simulink model "SeriesPHEV_New_Test2"  (R2018a)
settings: Solver=ode4  StartTime=0.0  StopTime=1367  FixedStep=0.01  RelTol=1e-3  EnableMultiTasking=on
undefined symbols (not defined in the file): cells, Eff, engine_rad, ES_dem, FDR, ftp, GT, InitialSOC, mdot, MG_dem, MGS, MT, P_ice, P_ice_dem, Regen, SOC_ICE, T_dem, tau_engine, throttle, time, Torq
settings Model: Creator=Administrator  LastModifiedBy=user2
settings DataIOCC: LimitDataPoints=on  SaveFormat=Array  SignalLoggingSaveFormat=ModelDataLogs
settings OptimizationCC: ExpressionDepthLimit=2147483647  LifeSpan=inf
settings DebuggingCC: UnderspecifiedInitializationDetection=Classic  MergeDetectMultiDrivingBlocksExec=none  SolverPrmCheckMsg=warning  FcnCallInpInsideContextMsg=warning  StateNameClashWarn=warning  SFUnexpectedBacktrackingDiag=warning  SFNoUnconditionalDefaultTransitionDiag=warning  SFExecutionAtInitializationDiag=none
settings HardwareCC: ProdBitPerPointer=32  ProdBitPerSizeT=32  ProdBitPerPtrDiffT=32  ProdLargestAtomicFloat=None  ProdIntDivRoundTo=Undefined  ProdEndianess=Unspecified  ProdWordSize=32  ProdHWDeviceType=32-bit Generic
settings ModelReferenceCC: PropagateSignalLabelsOutOfModel=off
settings CodeAppCC: StateflowObjectComments=on
settings GRTTargetCC: TargetLangStandard=C89/C90 (ANSI)  GeneratePreprocessorConditionals=Disable all  CombineOutputUpdateFcns=off  GRTInterface=on
settings ConfigComp: CovMetricSettings=dw  CovHtmlReporting=on  CovSaveCumulativeToWorkspaceVar=on  CovSaveSingleToWorkspaceVar=on  CovExternalEMLEnable=off

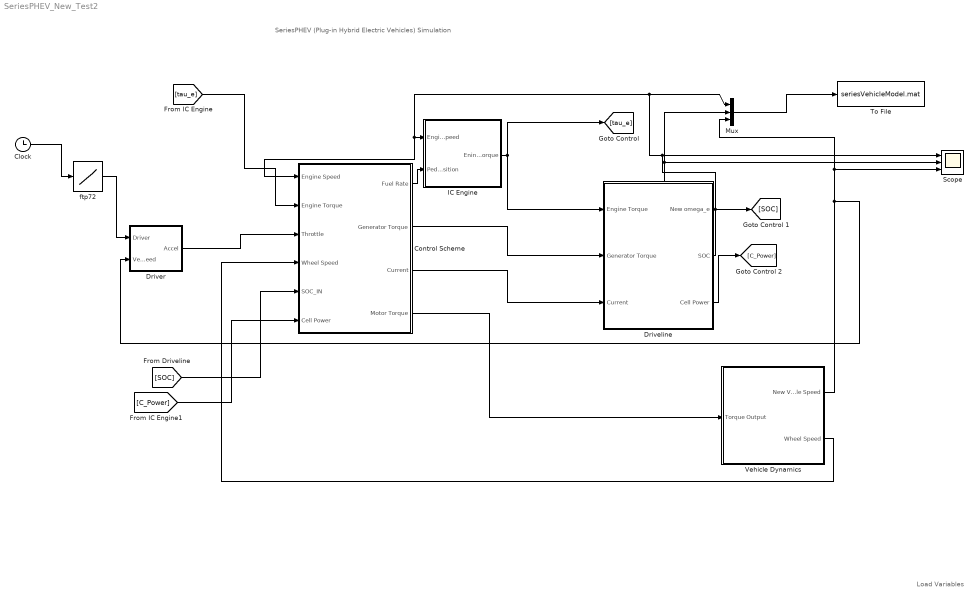
== system SeriesPHEV_New_Test2 ==
  note: SeriesPHEV (Plug-in Hybrid Electric Vehicles) Simulation
  note: Load Variables
  Clock : Clock
      settings: Decimation=100
  Control Scheme : Subsystem
  Driveline : Subsystem
  Driver : Subsystem
  IC Engine : Subsystem
  Mux : Mux  Inputs=3
  Scope : Scope  NumInputPorts=3
  To File : ToFile  Filename=seriesVehicleModel.mat  MatrixName=dynamics
  Vehicle Dynamics : Subsystem
  ftp72 : Lookup_n-D  NumberOfTableDimensions=1  BreakpointsForDimension1=time  Table=ftp  RndMeth=Simplest  InputSameDT=on
  wires:
  Mux/1 -> To File/1
  Driver/1(Accel) -> Control Scheme/3(Throttle)
  [SOC] -> Control Scheme/5(SOC_IN)
  Control Scheme/1(Fuel Rate) -> IC Engine/2(Pedal Position)
  IC Engine/1(Eninge Torque) -> [tau_e], Driveline/1(Engine Torque)
  Control Scheme/2(Generator Torque) -> Driveline/2(Generator Torque)
  Driveline/1(New omega_e) -> Mux/1, Control Scheme/1(Engine Speed), IC Engine/1(Engine Speed), Scope/1
  [tau_e] -> Control Scheme/2(Engine Torque)
  Vehicle Dynamics/1(New Vehicle Speed) -> Mux/3, Scope/3, Driver/2(Vehicle Speed)
  Vehicle Dynamics/2(Wheel Speed) -> Control Scheme/4(Wheel Speed)
  ftp72/1 -> Driver/1(Driver)
  Clock/1 -> ftp72/1
  Control Scheme/4(Motor Torque) -> Vehicle Dynamics/1(Torque Output)
  Driveline/2(SOC) -> Mux/2, Scope/2, [SOC]
  Control Scheme/3(Current) -> Driveline/3(Current)
  [C_Power] -> Control Scheme/6(Cell Power)
  Driveline/3(Cell Power) -> [C_Power]

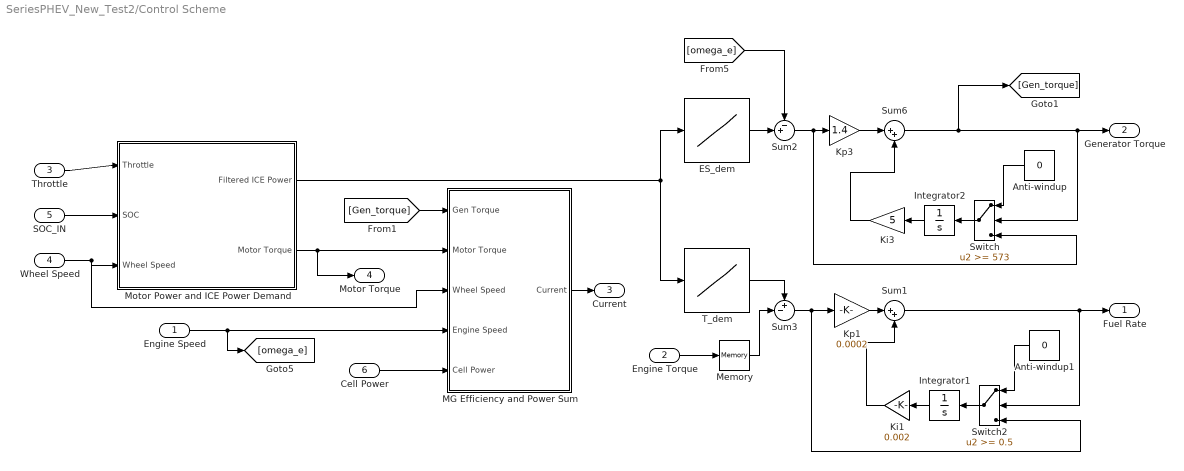
== system SeriesPHEV_New_Test2/Control Scheme ==
  Engine Speed : Inport
  Engine Torque : Inport  Port=2
  Throttle : Inport  Port=3
  Wheel Speed : Inport  Port=4
  SOC_IN : Inport  Port=5
  Cell Power : Inport  Port=6
  Anti-windup : Constant  Value=0
  Anti-windup1 : Constant  Value=0
  ES_dem : Lookup_n-D  NumberOfTableDimensions=1  BreakpointsForDimension1=P_ice  Table=ES_dem  RndMeth=Simplest  InputSameDT=on
  Integrator1 : Integrator
  Integrator2 : Integrator
  Ki1 : Gain  Gain=0.002
  Ki3 : Gain  Gain=5
  Kp1 : Gain  Gain=0.0002
  Kp3 : Gain  Gain=1.4
  MG Efficiency and Power Sum : Subsystem
  Memory : Memory  InheritSampleTime=on
  "Motor Power and ICE Power Demand " : Subsystem
  Sum1 : Sum  Inputs=|++
  Sum2 : Sum  Inputs=-+|
  Sum3 : Sum  Inputs=+-|
  Sum6 : Sum  Inputs=|++
  Switch : Switch  Threshold=573
  Switch2 : Switch  Threshold=0.5
  T_dem : Lookup_n-D  NumberOfTableDimensions=1  BreakpointsForDimension1=P_ice  Table=T_dem  RndMeth=Simplest  InputSameDT=on
  Fuel Rate : Outport
  Generator Torque : Outport  Port=2
  Current : Outport  Port=3
  Motor Torque : Outport  Port=4
  wires:
  ES_dem/1 -> Sum2/2
  T_dem/1 -> Sum3/1
  Engine Torque/1 -> Memory/1
  Kp3/1 -> Sum6/1
  Sum6/1 -> Generator Torque/1, Switch/2, [Gen_torque]
  Sum1/1 -> Fuel Rate/1, Switch2/2
  Memory/1 -> Sum3/2
  Switch/1 -> Integrator2/1
  Integrator2/1 -> Ki3/1
  Ki3/1 -> Sum6/2
  Sum2/1 -> Switch/3, Kp3/1
  Anti-windup/1 -> Switch/1
  Sum3/1 -> Kp1/1, Switch2/3
  Kp1/1 -> Sum1/1
  Switch2/1 -> Integrator1/1
  Integrator1/1 -> Ki1/1
  Ki1/1 -> Sum1/2
  Anti-windup1/1 -> Switch2/1
  MG Efficiency and Power Sum/1(Current) -> Current/1
  Cell Power/1 -> MG Efficiency and Power Sum/5(Cell Power)
  Throttle/1 -> "Motor Power and ICE Power Demand "/1(Throttle)
  SOC_IN/1 -> "Motor Power and ICE Power Demand "/2(SOC)
  Wheel Speed/1 -> "Motor Power and ICE Power Demand "/3(Wheel Speed), MG Efficiency and Power Sum/3(Wheel Speed)
  "Motor Power and ICE Power Demand "/2(Motor Torque) -> Motor Torque/1, MG Efficiency and Power Sum/2(Motor Torque)
  "Motor Power and ICE Power Demand "/1(Filtered ICE Power) -> T_dem/1, ES_dem/1
  [Gen_torque] -> MG Efficiency and Power Sum/1(Gen Torque)
  [omega_e] -> Sum2/1
  Engine Speed/1 -> MG Efficiency and Power Sum/4(Engine Speed), [omega_e]

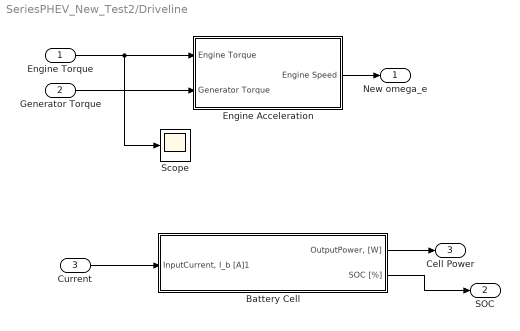
== system SeriesPHEV_New_Test2/Driveline ==
  Engine Torque : Inport
  Generator Torque : Inport  Port=2
  Current : Inport  Port=3
  Battery Cell : Subsystem
  Engine Acceleration : Subsystem
  Scope : Scope
  New omega_e : Outport
  SOC : Outport  Port=2
  Cell Power : Outport  Port=3
  wires:
  Engine Torque/1 -> Scope/1, Engine Acceleration/1(Engine Torque)
  Generator Torque/1 -> Engine Acceleration/2(Generator Torque)
  Engine Acceleration/1(Engine Speed) -> New omega_e/1
  Battery Cell/2(SOC [%]) -> SOC/1
  Current/1 -> Battery Cell/1("InputCurrent, I_b [A]1")
  Battery Cell/1("OutputPower, [W]") -> Cell Power/1

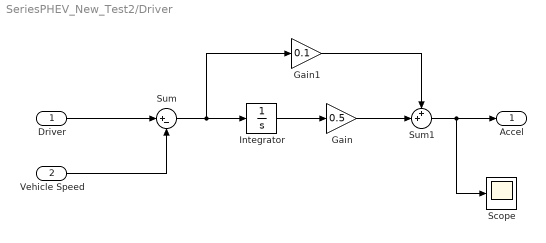
== system SeriesPHEV_New_Test2/Driver ==
  Driver : Inport
  Vehicle Speed : Inport  Port=2
  Gain : Gain  Gain=0.5
  Gain1 : Gain  Gain=0.1
  Integrator : Integrator
  Scope : Scope
  Sum : Sum  Inputs=|+-
  Sum1 : Sum  Inputs=++|
  Accel : Outport
  wires:
  Driver/1 -> Sum/1
  Vehicle Speed/1 -> Sum/2
  Sum/1 -> Integrator/1, Gain1/1
  Integrator/1 -> Gain/1
  Gain/1 -> Sum1/2
  Gain1/1 -> Sum1/1
  Sum1/1 -> Accel/1, Scope/1

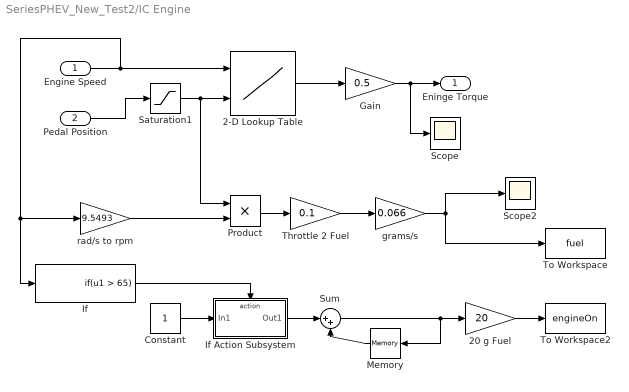
== system SeriesPHEV_New_Test2/IC Engine ==
  Engine Speed : Inport
  Pedal Position : Inport  Port=2
  2-D Lookup Table : Lookup_n-D  BreakpointsForDimension1=engine_rad  BreakpointsForDimension2=mdot  Table=tau_engine  RndMeth=Simplest  InputSameDT=on
  20 g Fuel : Gain  Gain=20
  Constant : Constant
  Gain : Gain  Gain=0.5
  If : If  IfExpression=u1 > 65  ShowElse=off
  If Action Subsystem : Subsystem  TreatAsAtomicUnit=on
  Memory : Memory
  Product : Product  RndMeth=Zero
  Saturation1 : Saturate  UpperLimit=0.4  LowerLimit=0
  Scope : Scope
  Scope2 : Scope
  Sum : Sum  Inputs=|++
  Throttle 2 Fuel : Gain  Gain=0.1
  To Workspace : ToWorkspace  VariableName=fuel  SampleTime=-1
      settings: Decimation=100
  To Workspace2 : ToWorkspace  VariableName=engineOn  SampleTime=-1
      settings: Decimation=100
  grams/s : Gain  Gain=0.066
  rad/s to rpm : Gain  Gain=9.5493
  Eninge Torque : Outport
  wires:
  Engine Speed/1 -> 2-D Lookup Table/1, rad/s to rpm/1, If/1
  Pedal Position/1 -> Saturation1/1
  Saturation1/1 -> Product/1, 2-D Lookup Table/2
  2-D Lookup Table/1 -> Gain/1
  Gain/1 -> Eninge Torque/1, Scope/1
  rad/s to rpm/1 -> Product/2
  grams/s/1 -> Scope2/1, To Workspace/1
  Memory/1 -> Sum/2
  If/1 -> If Action Subsystem/Action
  Constant/1 -> If Action Subsystem/1(In1)
  Sum/1 -> Memory/1, 20 g Fuel/1
  If Action Subsystem/1(Out1) -> Sum/1
  20 g Fuel/1 -> To Workspace2/1
  Throttle 2 Fuel/1 -> grams/s/1
  Product/1 -> Throttle 2 Fuel/1

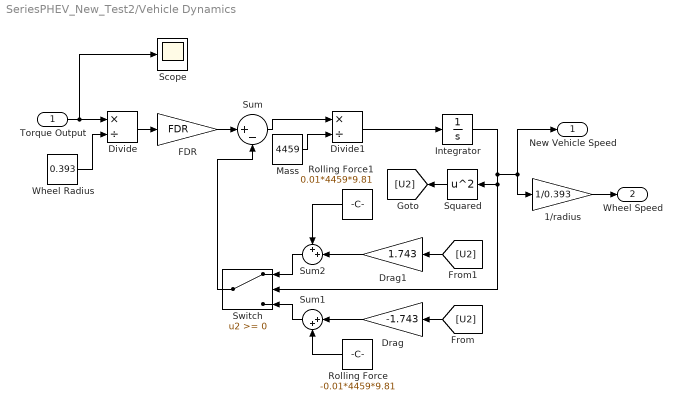
== system SeriesPHEV_New_Test2/Vehicle Dynamics ==
  Torque Output : Inport
  1/radius : Gain  Gain=1/0.393
  Divide : Product  Inputs=*/
  Divide1 : Product  Inputs=*/
  Drag : Gain  Gain=-1.743
  Drag1 : Gain  Gain=1.743
  FDR : Gain  Gain=FDR
  Integrator : Integrator
  Mass : Constant  Value=4459
  Rolling Force : Constant  Value=-0.01*4459*9.81
  Rolling Force1 : Constant  Value=0.01*4459*9.81
  Scope : Scope
  Squared : Math  Operator=square  SaturateOnIntegerOverflow=on
  Sum : Sum  Inputs=|+-
  Sum1 : Sum  Inputs=|++
  Sum2 : Sum  Inputs=++|
  Switch : Switch
  Wheel Radius : Constant  Value=0.393
  New Vehicle Speed : Outport
  Wheel Speed : Outport  Port=2
  wires:
  Torque Output/1 -> Scope/1, Divide/1
  Wheel Radius/1 -> Divide/2
  Divide/1 -> FDR/1
  1/radius/1 -> Wheel Speed/1
  Sum/1 -> Divide1/1
  Mass/1 -> Divide1/2
  Divide1/1 -> Integrator/1
  Integrator/1 -> 1/radius/1, New Vehicle Speed/1, Squared/1, Switch/2
  FDR/1 -> Sum/1
  Squared/1 -> [U2]
  Drag/1 -> Sum1/1
  Rolling Force/1 -> Sum1/2
  [U2] -> Drag/1
  Sum1/1 -> Switch/3
  [U2] -> Drag1/1
  Rolling Force1/1 -> Sum2/1
  Drag1/1 -> Sum2/2
  Sum2/1 -> Switch/1
  Switch/1 -> Sum/2

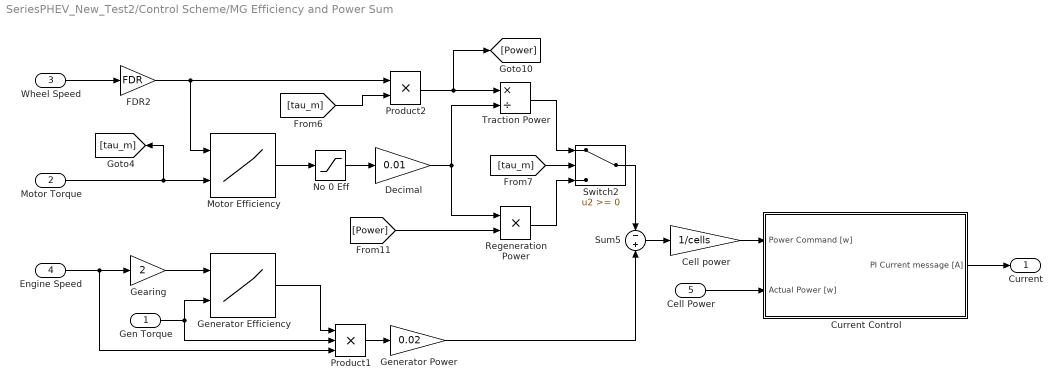
== system SeriesPHEV_New_Test2/Control Scheme/MG Efficiency and Power Sum ==
  Gen Torque : Inport
  Motor Torque : Inport  Port=2
  Wheel Speed : Inport  Port=3
  Engine Speed : Inport  Port=4
  Cell Power : Inport  Port=5
  Cell power : Gain  Gain=1/cells
  Current Control : Subsystem
  Decimal : Gain  Gain=0.01
  FDR2 : Gain  Gain=FDR
  Gearing : Gain  Gain=2
  Generator Power : Gain  Gain=0.02
  Generator Efficiency : Lookup_n-D  BreakpointsForDimension1=MGS  BreakpointsForDimension2=GT  Table=Eff  RndMeth=Simplest  InputSameDT=on
  Motor Efficiency : Lookup_n-D  BreakpointsForDimension1=MGS  BreakpointsForDimension2=MT  Table=Eff  RndMeth=Simplest  InputSameDT=on
  No 0 Eff : Saturate  UpperLimit=100  LowerLimit=0.001
  Product1 : Product  Inputs=3  RndMeth=Zero
  Product2 : Product  RndMeth=Zero
  Regeneration Power : Product  RndMeth=Zero
  Sum5 : Sum  Inputs=-+
  Switch2 : Switch
  Traction Power : Product  Inputs=*/
  Current : Outport
  wires:
  Gearing/1 -> Generator Efficiency/1
  Generator Efficiency/1 -> Product1/1
  Gen Torque/1 -> Product1/2, Generator Efficiency/2
  Product1/1 -> Generator Power/1
  Motor Efficiency/1 -> No 0 Eff/1
  [tau_m] -> Product2/2
  Product2/1 -> [Power], Traction Power/1
  Generator Power/1 -> Sum5/2
  Sum5/1 -> Cell power/1
  FDR2/1 -> Motor Efficiency/1, Product2/1
  No 0 Eff/1 -> Decimal/1
  Decimal/1 -> Regeneration Power/1, Traction Power/2
  [tau_m] -> Switch2/2
  Switch2/1 -> Sum5/1
  Regeneration Power/1 -> Switch2/3
  Traction Power/1 -> Switch2/1
  [Power] -> Regeneration Power/2
  Engine Speed/1 -> Product1/3, Gearing/1
  Motor Torque/1 -> [tau_m], Motor Efficiency/2
  Wheel Speed/1 -> FDR2/1
  Current Control/1(PI Current message [A]) -> Current/1
  Cell power/1 -> Current Control/1(Power Command [w])
  Cell Power/1 -> Current Control/2(Actual Power [w])

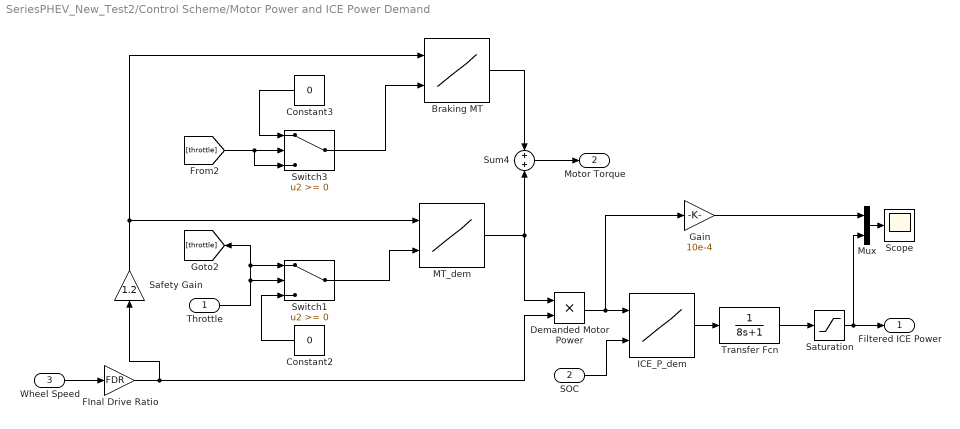
== system SeriesPHEV_New_Test2/Control Scheme/Motor Power and ICE Power Demand  ==
  Throttle : Inport
  SOC : Inport  Port=2
  Wheel Speed : Inport  Port=3
  Braking MT : Lookup_n-D  BreakpointsForDimension1=MGS  BreakpointsForDimension2=throttle  Table=Regen  RndMeth=Simplest  InputSameDT=on
  Constant2 : Constant  Value=0
  Constant3 : Constant  Value=0
  Demanded Motor Power : Product  RndMeth=Zero
  FInal Drive Ratio : Gain  Gain=FDR
  Gain : Gain  Gain=10e-4
  ICE_P_dem : Lookup_n-D  BreakpointsForDimension1=MG_dem  BreakpointsForDimension2=SOC_ICE  Table=P_ice_dem  RndMeth=Simplest  InputSameDT=on
  MT_dem : Lookup_n-D  BreakpointsForDimension1=MGS  BreakpointsForDimension2=mdot  Table=Torq  RndMeth=Simplest  InputSameDT=on
  Mux : Mux  Inputs=2
  Safety Gain : Gain  Gain=1.2
  Saturation : Saturate  UpperLimit=88.74  LowerLimit=0
  Scope : Scope
  Sum4 : Sum
  Switch1 : Switch
  Switch3 : Switch
  Transfer Fcn : TransferFcn  Denominator=[8 1]
  Filtered ICE Power : Outport
  Motor Torque : Outport  Port=2
  wires:
  FInal Drive Ratio/1 -> Demanded Motor Power/2, Safety Gain/1
  Safety Gain/1 -> MT_dem/1, Braking MT/1
  Demanded Motor Power/1 -> Gain/1, ICE_P_dem/1
  Switch1/1 -> MT_dem/2
  Constant2/1 -> Switch1/3
  Constant3/1 -> Switch3/1
  [throttle] -> Switch3/2, Switch3/3
  Switch3/1 -> Braking MT/2
  Transfer Fcn/1 -> Saturation/1
  ICE_P_dem/1 -> Transfer Fcn/1
  Braking MT/1 -> Sum4/1
  MT_dem/1 -> Sum4/2, Demanded Motor Power/1
  Wheel Speed/1 -> FInal Drive Ratio/1
  Throttle/1 -> [throttle], Switch1/1, Switch1/2
  SOC/1 -> ICE_P_dem/2
  Saturation/1 -> Mux/2, Filtered ICE Power/1
  Sum4/1 -> Motor Torque/1
  Mux/1 -> Scope/1
  Gain/1 -> Mux/1

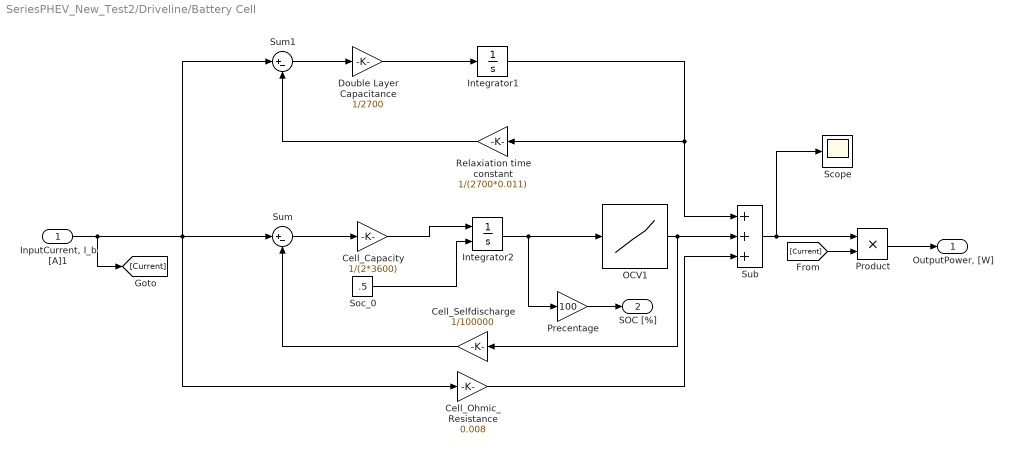
== system SeriesPHEV_New_Test2/Driveline/Battery Cell ==
  "InputCurrent, I_b [A]1" : Inport
  Cell_Capacity : Gain  Gain=1/(2*3600)
  Cell_Ohmic_Resistance : Gain  Gain=0.008
  Cell_Selfdischarge : Gain  Gain=1/100000
  Double Layer Capacitance : Gain  Gain=1/2700
  Integrator1 : Integrator
  Integrator2 : Integrator  InitialConditionSource=external  InitialCondition=InitialSOC
  OCV1 : Lookup_n-D  NumberOfTableDimensions=1  BreakpointsForDimension1=[0 0.1 0.2 0.3 0.4 0.5 0.6 0.7 0.8 0.9 1]  Table=[2.25 3.2 3.25 3.25 3.3 3.3 3.3 3.35 3.35 3.35 3.75]  RndMeth=Simplest  InputSameDT=on
  Precentage : Gain  Gain=100
  Product : Product  RndMeth=Zero
  Relaxiation time constant : Gain  Gain=1/(2700*0.011)
  Scope : Scope
  Soc_0 : Constant  Value=.5
  Sub : Sum  Inputs=+++
  Sum : Sum  Inputs=|+-
  Sum1 : Sum  Inputs=|+-
  "OutputPower, [W]" : Outport
  SOC [%] : Outport  Port=2
  wires:
  Integrator2/1 -> Precentage/1, OCV1/1
  OCV1/1 -> Cell_Selfdischarge/1, Sub/2
  "InputCurrent, I_b [A]1"/1 -> [Current], Sum1/1, Cell_Ohmic_Resistance/1, Sum/1
  Cell_Capacity/1 -> Integrator2/1
  Cell_Selfdischarge/1 -> Sum/2
  Integrator1/1 -> Relaxiation time constant/1, Sub/1
  Relaxiation time constant/1 -> Sum1/2
  Cell_Ohmic_Resistance/1 -> Sub/3
  Sub/1 -> Scope/1, Product/1
  Sum/1 -> Cell_Capacity/1
  Double Layer Capacitance/1 -> Integrator1/1
  Sum1/1 -> Double Layer Capacitance/1
  Soc_0/1 -> Integrator2/2
  [Current] -> Product/2
  Product/1 -> "OutputPower, [W]"/1
  Precentage/1 -> SOC [%]/1

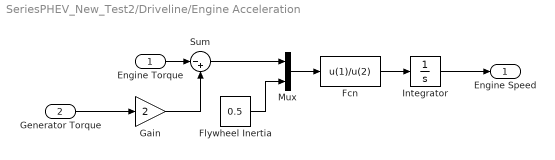
== system SeriesPHEV_New_Test2/Driveline/Engine Acceleration ==
  Engine Torque : Inport
  Generator Torque : Inport  Port=2
  Fcn : Fcn  Expr=u(1)/u(2)
  Flywheel Inertia : Constant  Value=0.5
  Gain : Gain  Gain=2
  Integrator : Integrator
  Mux : Mux  Inputs=2
  Sum : Sum  Inputs=|-+
  Engine Speed : Outport
  wires:
  Integrator/1 -> Engine Speed/1
  Engine Torque/1 -> Sum/1
  Sum/1 -> Mux/1
  Flywheel Inertia/1 -> Mux/2
  Mux/1 -> Fcn/1
  Fcn/1 -> Integrator/1
  Generator Torque/1 -> Gain/1
  Gain/1 -> Sum/2

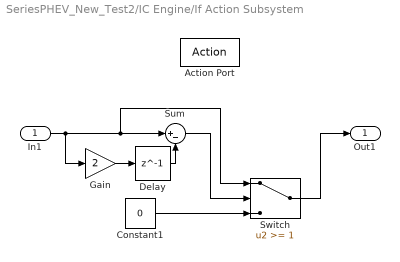
== system SeriesPHEV_New_Test2/IC Engine/If Action Subsystem ==
  In1 : Inport
  Action Port : ActionPort  InitializeStates=reset  ActionType=then
  Constant1 : Constant  Value=0
  Delay : Delay  DelayLength=1
  Gain : Gain  Gain=2
  Sum : Sum  Inputs=|+-
  Switch : Switch  Threshold=1
  Out1 : Outport  OutputWhenDisabled=reset  InitialOutput=[0]
  wires:
  Switch/1 -> Out1/1
  Constant1/1 -> Switch/3
  In1/1 -> Sum/1, Switch/1, Gain/1
  Delay/1 -> Sum/2
  Sum/1 -> Switch/2
  Gain/1 -> Delay/1

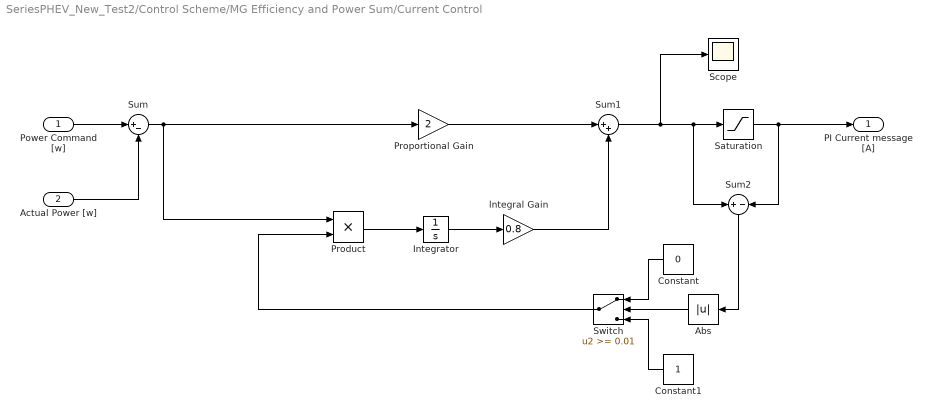
== system SeriesPHEV_New_Test2/Control Scheme/MG Efficiency and Power Sum/Current Control ==
  Power Command [w] : Inport
  Actual Power [w] : Inport  Port=2
  Abs : Abs
  Constant : Constant  Value=0
  Constant1 : Constant
  Integrator : Integrator
  Product : Product  RndMeth=Zero
  Proportional Gain : Gain  Gain=2
  Saturation : Saturate  UpperLimit=5  LowerLimit=-5  ZeroCross=off
  Scope : Scope
  Sum : Sum  Inputs=|+-
  Sum1 : Sum  Inputs=|++
  Sum2 : Sum  Inputs=+-
  Switch : Switch  Threshold=0.01
  lntegral Gain : Gain  Gain=0.8
  PI Current message [A] : Outport
  wires:
  Power Command [w]/1 -> Sum/1
  Actual Power [w]/1 -> Sum/2
  Sum/1 -> Proportional Gain/1, Product/1
  Proportional Gain/1 -> Sum1/1
  Sum1/1 -> Scope/1, Saturation/1, Sum2/1
  Saturation/1 -> PI Current message [A]/1, Sum2/2
  Integrator/1 -> lntegral Gain/1
  lntegral Gain/1 -> Sum1/2
  Sum2/1 -> Abs/1
  Abs/1 -> Switch/2
  Constant/1 -> Switch/1
  Constant1/1 -> Switch/3
  Switch/1 -> Product/2
  Product/1 -> Integrator/1
